simulink model "Analyse_parametres"  (R2020b)
settings: Solver=VariableStepAuto  StartTime=0.0  StopTime=10.0  RelTol=1e-3
values from neighbouring files (symbols this model uses):
  theta1 = 500    [Analyse_Robustesse.m]
  theta2 = -500    [Analyse_Robustesse.m]
undefined symbols (not defined in the file or in its folder): A_K1, Asous, B_K1, Bsous, C_K1, Csous, D_K1, Dsous
settings Model: Creator=Sandou  LastModifiedBy=Sandou

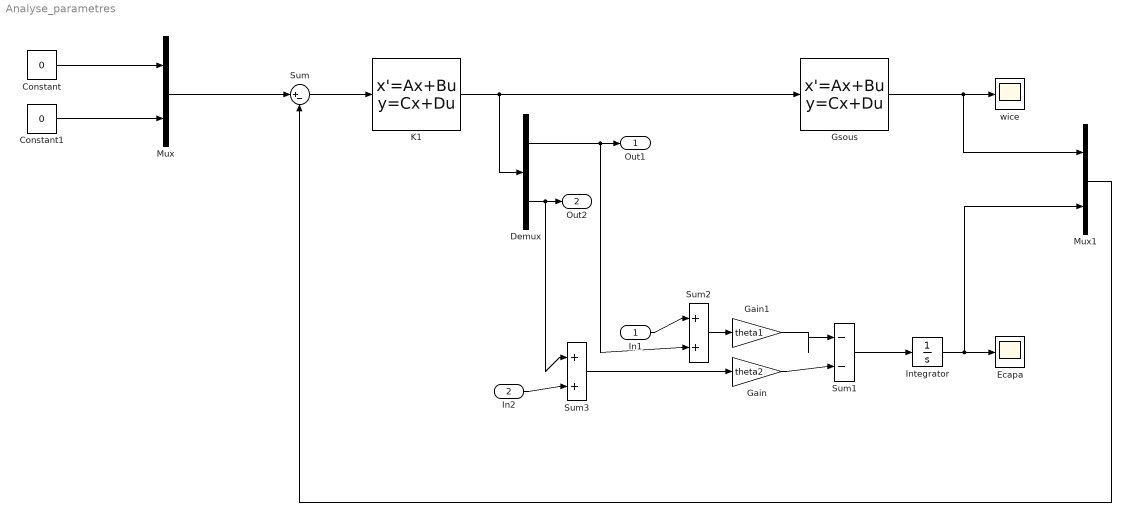
== system Analyse_parametres ==
  In1 : Inport
  In2 : Inport  Port=2
  Constant : Constant  Value=0
  Constant1 : Constant  Value=0
  Demux : Demux  Outputs=2
  Ecapa : Scope
  Gain : Gain  Gain=theta2
  Gain1 : Gain  Gain=theta1
  Gsous : StateSpace  A=Asous  B=Bsous  C=Csous  D=Dsous  InitialCondition=0
  Integrator : Integrator
  K1 : StateSpace  A=A_K1  B=B_K1  C=C_K1  D=D_K1  InitialCondition=0
  Mux : Mux  Inputs=2
  Mux1 : Mux  Inputs=2
  Sum : Sum  Inputs=|+-
  Sum1 : Sum  Inputs=|--
  Sum2 : Sum  Inputs=|++
  Sum3 : Sum  Inputs=|++
  wice : Scope
  Out1 : Outport
  Out2 : Outport  Port=2
  wires:
  Sum/1 -> K1/1
  Mux/1 -> Sum/1
  Constant/1 -> Mux/1
  Constant1/1 -> Mux/2
  K1/1 -> Demux/1, Gsous/1
  Gsous/1 -> Mux1/1, wice/1
  Integrator/1 -> Mux1/2, Ecapa/1
  Mux1/1 -> Sum/2
  Sum1/1 -> Integrator/1
  Gain/1 -> Sum1/2
  Gain1/1 -> Sum1/1
  Sum2/1 -> Gain1/1
  In1/1 -> Sum2/1
  Sum3/1 -> Gain/1
  In2/1 -> Sum3/2
  Demux/1 -> Sum2/2, Out1/1
  Demux/2 -> Out2/1, Sum3/1
